simulink model "full_system"  (R2023a)
settings: Solver=VariableStepAuto  StartTime=0.0  StopTime=10  RelTol=1e-3
undefined symbols (not defined in the file): graph_data, marker_data, node_data
settings Model: Creator=gabrielle  LastModifiedBy=gabrielle

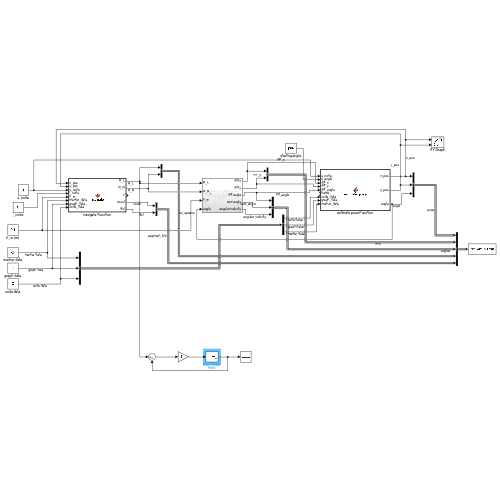
[thumbnail: Simulink's stored preview of the top-level diagram]
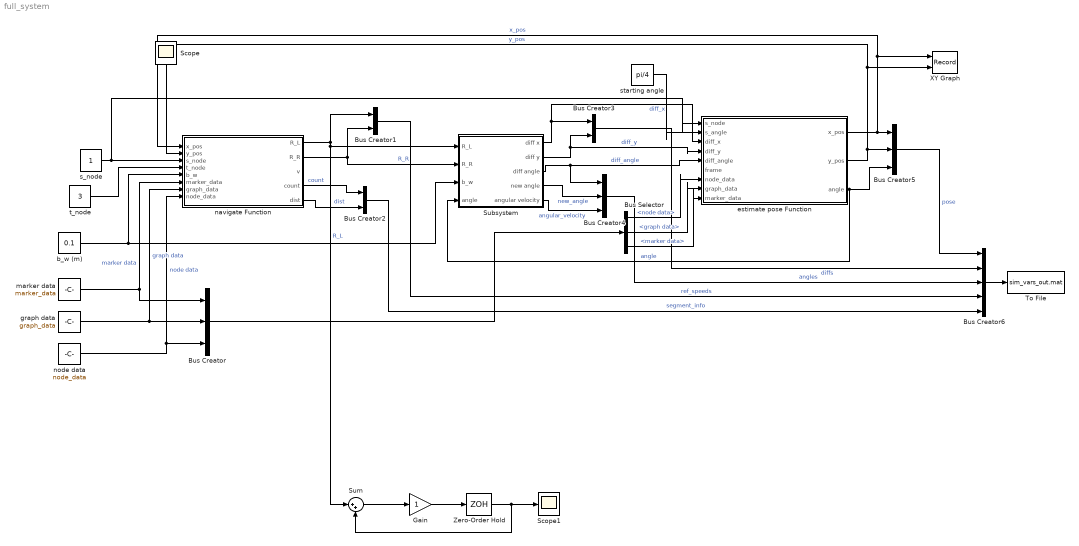
== system full_system ==
  Bus Creator : BusCreator  Inputs=3
  Bus Creator1 : BusCreator  Inputs=2
  Bus Creator2 : BusCreator  Inputs=2
  Bus Creator3 : BusCreator  Inputs=2
  Bus Creator4 : BusCreator  Inputs=3
  Bus Creator5 : BusCreator  Inputs=3
  Bus Creator6 : BusCreator  Inputs=5
  Bus Selector : BusSelector  OutputSignals=node data,graph data,marker data
  Gain : Gain
  Scope1 : Scope
  Subsystem : Subsystem
  Sum : Sum  Inputs=|++
  To File : ToFile  Filename=sim_vars_out.mat  SaveFormat=Timeseries
  XY Graph : Record  FileSettingsInternal="{\"entries\":[{\"content\":{\"excelSettings\":{\"content\":{},\"type\":\"Streamout.ExcelSettings\"}},\"type\":\"Streamout.FileSettingStorage\",\"uuid\":\"\"}],\"packageUris\":[\"http:\\/\\/schema.mathworks.com\\/mf0\\/streamout_blocks\\/R2020a\"],\"version\":\"1.0\"}"  Layout=[1 1]  SignalsInternal="{\"entries\":[{\"content\":{\"signals\":[{\"content\":{\"blockPath\":[],\"dimensions\":[1],\"domain\":\"\",\"lineColor\":\"#a2142f\",\"plots\":[1],\"port\":1,\"sid\":[\"\"],\"signalID\":945,\"signalName\":\"x_pos\"},\"type\":\"RecordBlkView.Signal\",\"uuid\":\"\"},{\"content\":{\"blockPath\":[],\"dimensions\":[1],\"domain\":\"\",\"lineColor\":\"#139fff\",\"plots\":[1],\"port\":2,\"sid\":[\"\"],\"signalID\":949,\"signalName\":\"y_pos\"},\"type\":\"RecordBlkView.Signal\",\"uuid\":\"\"}]},\"type\":\"RecordBlkView.InputSignals\",\"uuid\":\"\"}],\"packageUris\":[\"http:\\/\\/schema.mathworks.com\\/mf0\\/streamout_blocks\\/R2020a\"],\"version\":\"1.0\"}"  VisualizationBindings="{\"xyplotplugin\":{\"info\":[{\"series\":[{\"bindingParametersList\":[{\"parameter\":\"Y-Axis\",\"signalID\":949,\"signalName\":\"y_pos\"},{\"parameter\":\"X-Axis\",\"signalID\":945,\"signalName\":\"x_pos\"}],\"seriesID\":29316}],\"subplotID\":1}]}}"  CompatibilityTag=XY
  Zero-Order Hold : ZeroOrderHold  SampleTime=-1
  b_w (m) : Constant  Value=0.1
  estimate pose Function : MATLAB Function  TreatAsAtomicUnit=on
  graph data : Constant  Value=graph_data
  marker data : Constant  Value=marker_data  VectorParams1D=off
  navigate Function : MATLAB Function  TreatAsAtomicUnit=on
  node data : Constant  Value=node_data
  s_node : Constant
  starting angle : Constant  Value=pi/4
  t_node : Constant  Value=3
  Scope : Scope
  wires:
  b_w (m)/1 -> Subsystem/3(b_w), navigate Function/5(b_w)
  s_node/1 -> navigate Function/3(s_node), estimate pose Function/1(s_node)
  t_node/1 -> navigate Function/4(t_node)
  starting angle/1 -> estimate pose Function/2(s_angle)
  estimate pose Function/1(x_pos) -> Bus Creator5/1, XY Graph/1, navigate Function/1(x_pos)  "x_pos"
  estimate pose Function/2(y_pos) -> Bus Creator5/2, XY Graph/2, navigate Function/2(y_pos)  "y_pos"
  estimate pose Function/3(angle) -> Bus Creator5/3, Subsystem/4(angle)  "angle"
  marker data/1 -> Bus Creator/1, navigate Function/6(marker_data)  "marker data"
  graph data/1 -> Bus Creator/2, navigate Function/7(graph_data)  "graph data"
  node data/1 -> Bus Creator/3, navigate Function/8(node_data)  "node data"
  Bus Creator/1 -> Bus Selector/1
  Bus Selector/1 -> estimate pose Function/7(node_data)  "<node data>"
  Bus Selector/2 -> estimate pose Function/8(graph_data)  "<graph data>"
  Bus Selector/3 -> estimate pose Function/9(marker_data)  "<marker data>"
  navigate Function/1(R_L) -> Bus Creator1/1, Sum/1, Subsystem/1(R_L)  "R_L"
  navigate Function/2(R_R) -> Bus Creator1/2, Subsystem/2(R_R)  "R_R"
  Subsystem/1(diff x) -> estimate pose Function/3(diff_x), Bus Creator3/1  "diff_x"
  Subsystem/2(diff y) -> Bus Creator3/2, estimate pose Function/4(diff_y)  "diff_y"
  navigate Function/5(dist) -> Bus Creator2/2  "dist"
  Subsystem/3(diff angle) -> Bus Creator4/1, estimate pose Function/5(diff_angle)  "diff_angle"
  navigate Function/4(count) -> Bus Creator2/1  "count"
  Subsystem/4(new angle) -> Bus Creator4/2  "new_angle"
  Subsystem/5(angular velocity) -> Bus Creator4/3  "angular_velocity"
  Bus Creator5/1 -> Bus Creator6/1  "pose"
  Bus Creator3/1 -> Bus Creator6/2  "diffs"
  Bus Creator4/1 -> Bus Creator6/3  "angles"
  Bus Creator1/1 -> Bus Creator6/4  "ref_speeds"
  Bus Creator2/1 -> Bus Creator6/5  "segment_info"
  Bus Creator6/1 -> To File/1
  Sum/1 -> Gain/1
  Gain/1 -> Zero-Order Hold/1
  Zero-Order Hold/1 -> Sum/2, Scope1/1

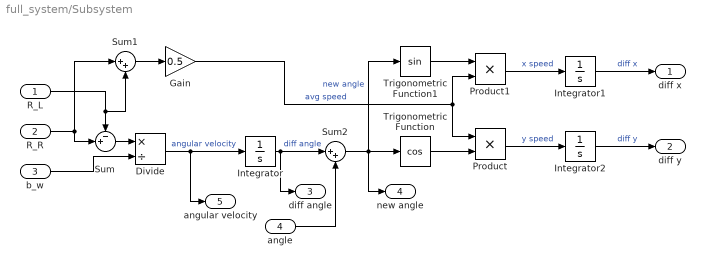
== system full_system/Subsystem ==
  R_L : Inport
  R_R : Inport  Port=2
  b_w : Inport  Port=3
  angle : Inport  Port=4
  Divide : Product  Inputs=*/
  Gain : Gain  Gain=0.5
  Integrator : Integrator
  Integrator1 : Integrator
  Integrator2 : Integrator
  Product : Product
  Product1 : Product
  Sum : Sum  Inputs=-+|
  Sum1 : Sum  Inputs=|++
  Sum2 : Sum  Inputs=|++
  Trigonometric Function : Trigonometry  Operator=cos
  Trigonometric Function1 : Trigonometry
  diff x : Outport
  diff y : Outport  Port=2
  diff angle : Outport  Port=3
  new angle : Outport  Port=4
  angular velocity : Outport  Port=5
  wires:
  b_w/1 -> Divide/2
  R_L/1 -> Sum/1, Sum1/2
  Trigonometric Function1/1 -> Product1/1
  Gain/1 -> Product/1, Product1/2  "avg speed"
  R_R/1 -> Sum/2, Sum1/1
  Product1/1 -> Integrator1/1  "x speed"
  Sum1/1 -> Gain/1
  Sum/1 -> Divide/1
  Trigonometric Function/1 -> Product/2
  Divide/1 -> angular velocity/1, Integrator/1  "angular velocity"
  Product/1 -> Integrator2/1  "y speed"
  Integrator/1 -> diff angle/1, Sum2/1  "diff angle"
  angle/1 -> Sum2/2
  Sum2/1 -> Trigonometric Function/1, Trigonometric Function1/1, new angle/1  "new angle"
  Integrator1/1 -> diff x/1  "diff x"
  Integrator2/1 -> diff y/1  "diff y"

== matlab function full_system/estimate pose Function ==
  settings: updateMethod=DISCRETE
  data: s_node input; s_angle input; x_pos output; diff_x input; diff_y input; diff_angle input; y_pos output; angle output; frame input; node_data input; graph_data input; marker_data input
function [x_pos, y_pos, angle] = estimate_pose(s_node, s_angle, diff_x, ...
    diff_y, diff_angle, frame, node_data, graph_data, marker_data)

persistent map;
persistent poseEsitmator;

gotMarker = 0;
marker_pose = [0; 0; 0];

if isempty(map)
    map =  assemble_map(node_data, graph_data, marker_data);
    %map = map.map_data;
end

if isempty(poseEsitmator)
    nd = map.nodes{s_node};
    s_pose = [nd.x_coord; nd.y_coord; s_angle];

    poseEsitmator = pose_estimator(map, s_pose);
end

% if ~isempty(frame)
%     [id, loc, pose, gotMarker] = find_markers(poseEsitmator, frame);
% 
%     if gotMarker==1
%         marker_pose = pose_from_marker(id, loc, pose);
%     end
% end

controlPose = pose_from_control(poseEsitmator, diff_x, diff_y, diff_angle);

poseEsitmator = update_pose(poseEsitmator, marker_pose, gotMarker, controlPose);
current_pose = get_current_pose(poseEsitmator);

x_pos = current_pose(1);
y_pos = current_pose(2);
angle = current_pose(3);

== matlab function full_system/navigate Function ==
  data: x_pos input; R_L output; R_R output; y_pos input; v output; count output; s_node input; t_node input; b_w input; marker_data input; graph_data input; node_data input; dist output
function [R_L, R_R, v, count, dist] = navigate(x_pos, y_pos, s_node, t_node, b_w, marker_data, graph_data, node_data)
persistent routePlanner;
persistent ref_signal;
persistent map;
persistent seg_count;
persistent stopped;

if isempty(stopped)
    stopped = 0;
end

%persistent path;
if stopped==0
    v = 0.4; %m/s
else
    v = 0;
end
max_dist = 0.2; %m 
brake_dist = 0.5; %m
stop_dist = 0.05; %m

if isempty(map)
    map =  assemble_map(node_data, graph_data, marker_data);
    %map = map.map_data;
end

if isempty(routePlanner)
    routePlanner = route_planner(map);
end

if isempty(ref_signal)
    [path, ~] = plot_route(routePlanner, s_node, t_node);
    ref_signal = convert_to_ref_array(routePlanner, path);
   % ref_signal = [0; 0; 4; 3; 0];
end

len_ref = size(ref_signal);
len_ref = len_ref(2);


if isempty(seg_count)
    seg_count = 1;
end


x_diff = ref_signal(3, seg_count) - x_pos; 
y_diff = ref_signal(4, seg_count) - y_pos; 
dist = sqrt(x_diff^2 + y_diff^2);

if (dist <= max_dist) && (seg_count < len_ref)
    seg_count = seg_count + 1;
end

if (dist <= brake_dist) && (seg_count == len_ref)
    mult = (dist - stop_dist)/(brake_dist - stop_dist);
    v = v*mult;

    if v<=0
        stopped = 1;
    end
end

R = ref_signal(5,seg_count);
if R==0
    R_L = v;
    R_R = v;
else
    % if R<=1
    %     v = v*abs(R);
    % end

    R_L = v*(1-(b_w/(2*R)));
    R_R = v*(1+(b_w/(2*R)));
end



count = seg_count;
